simulink model "Kinematic_Model_Simulink"  (R2022a)
settings: Solver=ode14x  StartTime=0.0  StopTime=0.7  FixedStep=0.0005  RelTol=1e-3
values from neighbouring files (symbols this model uses):
  a_joint = 160/180*pi    (= 2.79252680319)    [Kinematic_Model_Activation.m]    (also in Kinematic_Model_sweep_double.m; Kinematic_Model_sweep_single.m)
  C_damping = 10    [Kinematic_Model_Activation.m]    (also in Kinematic_Model_sweep_double.m; Kinematic_Model_sweep_single.m = 100)
  g = [0;0;-9.81]    [Kinematic_Model_Activation.m]    (also in Kinematic_Model_sweep_double.m; Kinematic_Model_sweep_single.m)
  k_cable = 1200    [Kinematic_Model_Activation.m]    (also in Kinematic_Model_sweep_single.m)
  k_joint = 35    [Kinematic_Model_Activation.m]    (also in Kinematic_Model_sweep_double.m; Kinematic_Model_sweep_single.m)
  l_cable = sqrt(6)/4*l_leg*sin(a_joint/2)*(1 - delta)    [Kinematic_Model_Activation.m]    (also in Kinematic_Model_sweep_double.m; Kinematic_Model_sweep_single.m)
  l_leg = 0.3    [Kinematic_Model_Activation.m]    (also in Kinematic_Model_sweep_double.m; Kinematic_Model_sweep_single.m)
  m_bar = m_leg/2    (= 0.331383847657)    [Kinematic_Model_Activation.m]    (also in Kinematic_Model_sweep_double.m; Kinematic_Model_sweep_single.m)
  mu_k = 0.35    [Kinematic_Model_Activation.m]    (also in Kinematic_Model_sweep_double.m; Kinematic_Model_sweep_single.m)
  mu_s = 0.45    [Kinematic_Model_Activation.m]    (also in Kinematic_Model_sweep_double.m; Kinematic_Model_sweep_single.m)
  nu_s = 0.2    [Kinematic_Model_Activation.m]    (also in Kinematic_Model_sweep_double.m; Kinematic_Model_sweep_single.m)
  T_damping = 1    [Kinematic_Model_Activation.m]    (also in Kinematic_Model_sweep_double.m; Kinematic_Model_sweep_single.m)
(part 1 of 2)
settings Model: Creator=LZY-ALIENWARE15  LastModifiedBy=S2974177
settings SolverCC: ExtrapolationOrder=3  AlgebraicLoopSolver=TrustRegion
settings DebuggingCC: UnconnectedInputMsg=warning  UnconnectedOutputMsg=warning  UnconnectedLineMsg=warning  SFMachineParentedDataDiag=warning  UnderSpecifiedDimensionMsg=warning
settings RTWCC: DLArmComputeVersion=19.05

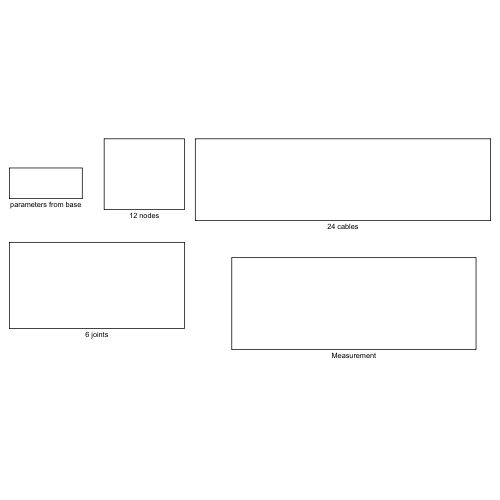
[thumbnail: Simulink's stored preview of the top-level diagram]
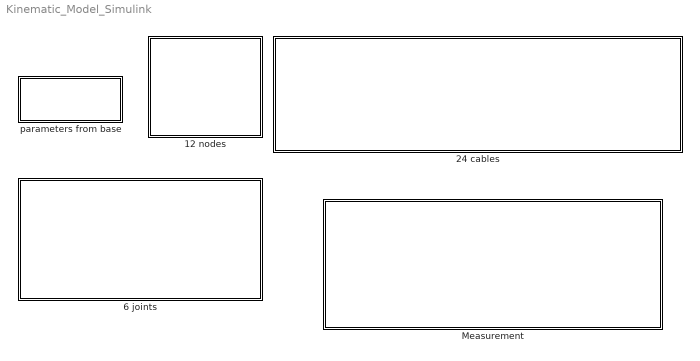
== system Kinematic_Model_Simulink ==
  "12 nodes " : Subsystem
  24 cables : Subsystem
  6 joints : Subsystem
  Measurement : Subsystem
  parameters from base : Subsystem

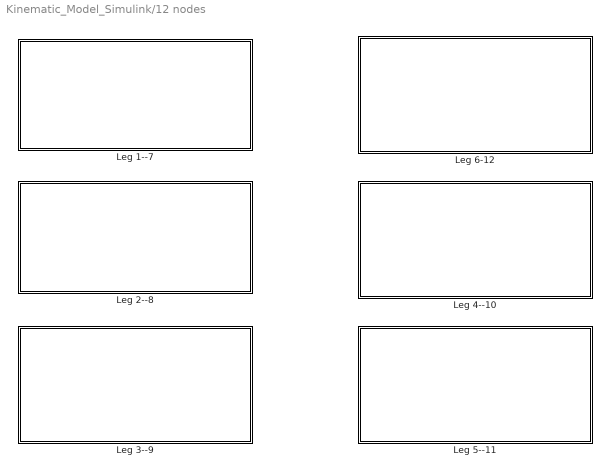
== system Kinematic_Model_Simulink/12 nodes  ==
  Leg 1--7 : Subsystem
  Leg 2--8 : Subsystem
  Leg 3--9 : Subsystem
  Leg 4--10 : Subsystem
  Leg 5--11 : Subsystem
  Leg 6-12 : Subsystem

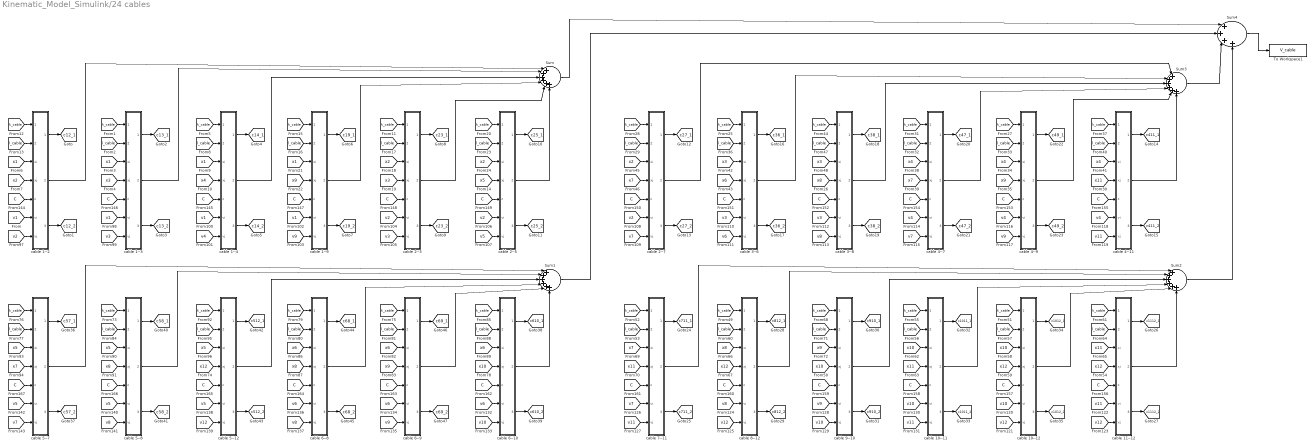
== system Kinematic_Model_Simulink/24 cables ==
  Sum{,1..3} (4 alike) : Sum  Inputs=|++++++
  Sum4 : Sum  Inputs=|++++
  To Workspace1 : ToWorkspace  VariableName=V_cable  SaveFormat=Timeseries  SampleTime=-1
  cable 1--2 : MATLAB Function  TreatAsAtomicUnit=on
  cable 1--3 : MATLAB Function  TreatAsAtomicUnit=on
  cable 1--4 : MATLAB Function  TreatAsAtomicUnit=on
  cable 1--9 : MATLAB Function  TreatAsAtomicUnit=on
  cable 10--11 : MATLAB Function  TreatAsAtomicUnit=on
  cable 10--12 : MATLAB Function  TreatAsAtomicUnit=on
  cable 11--12 : MATLAB Function  TreatAsAtomicUnit=on
  cable 2--3 : MATLAB Function  TreatAsAtomicUnit=on
  cable 2--5 : MATLAB Function  TreatAsAtomicUnit=on
  cable 2--7 : MATLAB Function  TreatAsAtomicUnit=on
  cable 3--6 : MATLAB Function  TreatAsAtomicUnit=on
  cable 3--8 : MATLAB Function  TreatAsAtomicUnit=on
  cable 4--11 : MATLAB Function  TreatAsAtomicUnit=on
  cable 4--7 : MATLAB Function  TreatAsAtomicUnit=on
  cable 4--9 : MATLAB Function  TreatAsAtomicUnit=on
  cable 5--12 : MATLAB Function  TreatAsAtomicUnit=on
  cable 5--7 : MATLAB Function  TreatAsAtomicUnit=on
  cable 5--8 : MATLAB Function  TreatAsAtomicUnit=on
  cable 6--10 : MATLAB Function  TreatAsAtomicUnit=on
  cable 6--8 : MATLAB Function  TreatAsAtomicUnit=on
  cable 6--9 : MATLAB Function  TreatAsAtomicUnit=on
  cable 7--11 : MATLAB Function  TreatAsAtomicUnit=on
  cable 8--12 : MATLAB Function  TreatAsAtomicUnit=on
  cable 9--10 : MATLAB Function  TreatAsAtomicUnit=on
  tag scope: c1011_1=global, c1011_2=global, c1012_1=global, c1012_2=global, c1112_1=global, c1112_2=global, c12_1=global, c12_2=global, c13_1=global, c13_2=global, c14_1=global, c14_2=global, c19_1=global, c19_2=global, c23_1=global, c23_2=global, c25_1=global, c25_2=global, c27_1=global, c27_2=global, c36_1=global, c36_2=global, c38_1=global, c38_2=global, c411_1=global, c411_2=global, c47_1=global, c47_2=global, c49_1=global, c49_2=global, c512_1=global, c512_2=global, c57_1=global, c57_2=global, c58_1=global, c58_2=global, c610_1=global, c610_2=global, c68_1=global, c68_2=global, c69_1=global, c69_2=global, c711_1=global, c711_2=global, c812_1=global, c812_2=global, c910_1=global, c910_2=global
  wires:
  [k_cable] -> cable 1--2/1(k_cable)
  [x1] -> cable 1--2/3(xi)
  [x2] -> cable 1--2/4(xj)
  cable 1--2/1(out_i) -> [c12_1]
  cable 1--2/3(out_j) -> [c12_2]
  [l_cable] -> cable 1--2/2(l_cable)
  [l_cable] -> cable 1--3/2(l_cable)
  [x1] -> cable 1--3/3(xi)
  [x3] -> cable 1--3/4(xj)
  cable 1--3/3(out_j) -> [c13_2]
  [k_cable] -> cable 1--3/1(k_cable)
  cable 1--3/1(out_i) -> [c13_1]
  [l_cable] -> cable 1--4/2(l_cable)
  [x1] -> cable 1--4/3(xi)
  [x4] -> cable 1--4/4(xj)
  cable 1--4/3(out_j) -> [c14_2]
  [k_cable] -> cable 1--4/1(k_cable)
  cable 1--4/1(out_i) -> [c14_1]
  [l_cable] -> cable 2--3/2(l_cable)
  [k_cable] -> cable 2--5/1(k_cable)
  cable 2--5/1(out_i) -> [c25_1]
  [x2] -> cable 2--5/3(xi)
  cable 2--5/3(out_j) -> [c25_2]
  cable 2--3/1(out_i) -> [c23_1]
  cable 2--3/3(out_j) -> [c23_2]
  [x3] -> cable 2--3/4(xj)
  [x1] -> cable 1--9/3(xi)
  [l_cable] -> cable 1--9/2(l_cable)
  [l_cable] -> cable 2--5/2(l_cable)
  [x9] -> cable 1--9/4(xj)
  [k_cable] -> cable 1--9/1(k_cable)
  [x2] -> cable 2--3/3(xi)
  cable 1--9/3(out_j) -> [c19_2]
  [k_cable] -> cable 2--3/1(k_cable)
  cable 1--9/1(out_i) -> [c19_1]
  [x5] -> cable 2--5/4(xj)
  [l_cable] -> cable 3--6/2(l_cable)
  [k_cable] -> cable 3--8/1(k_cable)
  cable 3--8/1(out_i) -> [c38_1]
  cable 3--8/3(out_j) -> [c38_2]
  cable 3--6/1(out_i) -> [c36_1]
  cable 3--6/3(out_j) -> [c36_2]
  [x6] -> cable 3--6/4(xj)
  [x7] -> cable 4--7/4(xj)
  [l_cable] -> cable 4--7/2(l_cable)
  [x4] -> cable 4--7/3(xi)
  [x9] -> cable 4--9/4(xj)
  cable 4--9/3(out_j) -> [c49_2]
  cable 4--11/3(out_j) -> [c411_2]
  [x4] -> cable 4--11/3(xi)
  [x11] -> cable 4--11/4(xj)
  cable 4--9/1(out_i) -> [c49_1]
  cable 4--7/1(out_i) -> [c47_1]
  [k_cable] -> cable 4--9/1(k_cable)
  cable 4--7/3(out_j) -> [c47_2]
  [k_cable] -> cable 4--7/1(k_cable)
  [x4] -> cable 4--9/3(xi)
  [x7] -> cable 2--7/4(xj)
  cable 2--7/3(out_j) -> [c27_2]
  [x3] -> cable 3--6/3(xi)
  [k_cable] -> cable 2--7/1(k_cable)
  [l_cable] -> cable 4--11/2(l_cable)
  cable 4--11/1(out_i) -> [c411_1]
  [x3] -> cable 3--8/3(xi)
  cable 2--7/1(out_i) -> [c27_1]
  [k_cable] -> cable 3--6/1(k_cable)
  [x8] -> cable 3--8/4(xj)
  [k_cable] -> cable 4--11/1(k_cable)
  [x2] -> cable 2--7/3(xi)
  [l_cable] -> cable 2--7/2(l_cable)
  [l_cable] -> cable 3--8/2(l_cable)
  [l_cable] -> cable 4--9/2(l_cable)
  [l_cable] -> cable 8--12/2(l_cable)
  [k_cable] -> cable 9--10/1(k_cable)
  cable 9--10/1(out_i) -> [c910_1]
  cable 9--10/3(out_j) -> [c910_2]
  cable 8--12/1(out_i) -> [c812_1]
  cable 8--12/3(out_j) -> [c812_2]
  [x12] -> cable 8--12/4(xj)
  [x11] -> cable 10--11/4(xj)
  [l_cable] -> cable 10--11/2(l_cable)
  [x10] -> cable 10--11/3(xi)
  [x12] -> cable 10--12/4(xj)
  cable 10--12/3(out_j) -> [c1012_2]
  cable 11--12/3(out_j) -> [c1112_2]
  [x11] -> cable 11--12/3(xi)
  [x12] -> cable 11--12/4(xj)
  cable 10--12/1(out_i) -> [c1012_1]
  cable 10--11/1(out_i) -> [c1011_1]
  [k_cable] -> cable 10--12/1(k_cable)
  cable 10--11/3(out_j) -> [c1011_2]
  [k_cable] -> cable 10--11/1(k_cable)
  [x10] -> cable 10--12/3(xi)
  [x11] -> cable 7--11/4(xj)
  cable 7--11/3(out_j) -> [c711_2]
  [x8] -> cable 8--12/3(xi)
  [k_cable] -> cable 7--11/1(k_cable)
  [l_cable] -> cable 11--12/2(l_cable)
  cable 11--12/1(out_i) -> [c1112_1]
  [x9] -> cable 9--10/3(xi)
  cable 7--11/1(out_i) -> [c711_1]
  [k_cable] -> cable 8--12/1(k_cable)
  [x10] -> cable 9--10/4(xj)
  [k_cable] -> cable 11--12/1(k_cable)
  [x7] -> cable 7--11/3(xi)
  [l_cable] -> cable 7--11/2(l_cable)
  [l_cable] -> cable 9--10/2(l_cable)
  [l_cable] -> cable 10--12/2(l_cable)
  [l_cable] -> cable 5--8/2(l_cable)
  [k_cable] -> cable 5--12/1(k_cable)
  cable 5--12/1(out_i) -> [c512_1]
  cable 5--12/3(out_j) -> [c512_2]
  cable 5--8/1(out_i) -> [c58_1]
  cable 5--8/3(out_j) -> [c58_2]
  [x8] -> cable 5--8/4(xj)
  [x8] -> cable 6--8/4(xj)
  [l_cable] -> cable 6--8/2(l_cable)
  [x6] -> cable 6--8/3(xi)
  [x9] -> cable 6--9/4(xj)
  cable 6--9/3(out_j) -> [c69_2]
  cable 6--10/3(out_j) -> [c610_2]
  [x6] -> cable 6--10/3(xi)
  [x10] -> cable 6--10/4(xj)
  cable 6--9/1(out_i) -> [c69_1]
  cable 6--8/1(out_i) -> [c68_1]
  [k_cable] -> cable 6--9/1(k_cable)
  cable 6--8/3(out_j) -> [c68_2]
  [k_cable] -> cable 6--8/1(k_cable)
  [x6] -> cable 6--9/3(xi)
  [x7] -> cable 5--7/4(xj)
  cable 5--7/3(out_j) -> [c57_2]
  [x5] -> cable 5--8/3(xi)
  [k_cable] -> cable 5--7/1(k_cable)
  [l_cable] -> cable 6--10/2(l_cable)
  cable 6--10/1(out_i) -> [c610_1]
  [x5] -> cable 5--12/3(xi)
  cable 5--7/1(out_i) -> [c57_1]
  [k_cable] -> cable 5--8/1(k_cable)
  [x12] -> cable 5--12/4(xj)
  [k_cable] -> cable 6--10/1(k_cable)
  [x5] -> cable 5--7/3(xi)
  [l_cable] -> cable 5--7/2(l_cable)
  [l_cable] -> cable 5--12/2(l_cable)
  [l_cable] -> cable 6--9/2(l_cable)
  cable 1--2/2(E_cable) -> Sum/1
  cable 10--11/2(E_cable) -> Sum2/4
  cable 9--10/2(E_cable) -> Sum2/3
  cable 10--12/2(E_cable) -> Sum2/5
  cable 11--12/2(E_cable) -> Sum2/6
  cable 8--12/2(E_cable) -> Sum2/2
  cable 7--11/2(E_cable) -> Sum2/1
  cable 6--10/2(E_cable) -> Sum1/6
  cable 6--9/2(E_cable) -> Sum1/5
  cable 6--8/2(E_cable) -> Sum1/4
  cable 5--12/2(E_cable) -> Sum1/3
  cable 5--8/2(E_cable) -> Sum1/2
  cable 5--7/2(E_cable) -> Sum1/1
  cable 1--3/2(E_cable) -> Sum/2
  cable 1--4/2(E_cable) -> Sum/3
  cable 1--9/2(E_cable) -> Sum/4
  cable 2--3/2(E_cable) -> Sum/5
  cable 2--5/2(E_cable) -> Sum/6
  cable 2--7/2(E_cable) -> Sum3/1
  cable 3--6/2(E_cable) -> Sum3/2
  cable 3--8/2(E_cable) -> Sum3/3
  cable 4--7/2(E_cable) -> Sum3/4
  cable 4--9/2(E_cable) -> Sum3/5
  cable 4--11/2(E_cable) -> Sum3/6
  Sum3/1 -> Sum4/3
  Sum2/1 -> Sum4/4
  Sum1/1 -> Sum4/2
  Sum/1 -> Sum4/1
  Sum4/1 -> To Workspace1/1
  [v1] -> cable 1--2/6(vi)
  [v2] -> cable 1--2/7(vj)
  [v4] -> cable 1--4/7(vj)
  [v1] -> cable 1--4/6(vi)
  [v1] -> cable 1--9/6(vi)
  [v9] -> cable 1--9/7(vj)
  [v1] -> cable 1--3/6(vi)
  [v3] -> cable 1--3/7(vj)
  [v2] -> cable 2--3/6(vi)
  [v3] -> cable 2--3/7(vj)
  [v2] -> cable 2--5/6(vi)
  [v5] -> cable 2--5/7(vj)
  [v2] -> cable 2--7/6(vi)
  [v7] -> cable 2--7/7(vj)
  [v3] -> cable 3--6/6(vi)
  [v6] -> cable 3--6/7(vj)
  [v3] -> cable 3--8/6(vi)
  [v8] -> cable 3--8/7(vj)
  [v4] -> cable 4--7/6(vi)
  [v7] -> cable 4--7/7(vj)
  [v4] -> cable 4--9/6(vi)
  [v9] -> cable 4--9/7(vj)
  [v4] -> cable 4--11/6(vi)
  [v11] -> cable 4--11/7(vj)
  [v10] -> cable 10--12/6(vi)
  [v12] -> cable 10--12/7(vj)
  [v11] -> cable 11--12/6(vi)
  [v12] -> cable 11--12/7(vj)
  [v8] -> cable 8--12/6(vi)
  [v12] -> cable 8--12/7(vj)
  [v7] -> cable 7--11/6(vi)
  [v11] -> cable 7--11/7(vj)
  [v9] -> cable 9--10/6(vi)
  [v10] -> cable 9--10/7(vj)
  [v10] -> cable 10--11/6(vi)
  [v11] -> cable 10--11/7(vj)
  [v6] -> cable 6--10/6(vi)
  [v10] -> cable 6--10/7(vj)
  [v6] -> cable 6--9/6(vi)
  [v9] -> cable 6--9/7(vj)
  [v6] -> cable 6--8/6(vi)
  [v8] -> cable 6--8/7(vj)
  [v5] -> cable 5--12/6(vi)
  [v12] -> cable 5--12/7(vj)
  [v5] -> cable 5--8/6(vi)
  [v8] -> cable 5--8/7(vj)
  [v5] -> cable 5--7/6(vi)
  [v7] -> cable 5--7/7(vj)
  [C] -> cable 1--2/5(c)
  [C] -> cable 1--4/5(c)
  [C] -> cable 1--3/5(c)
  [C] -> cable 1--9/5(c)
  [C] -> cable 2--3/5(c)
  [C] -> cable 2--5/5(c)
  [C] -> cable 2--7/5(c)
  [C] -> cable 3--6/5(c)
  [C] -> cable 3--8/5(c)
  [C] -> cable 4--9/5(c)
  [C] -> cable 4--7/5(c)
  [C] -> cable 4--11/5(c)
  [C] -> cable 11--12/5(c)
  [C] -> cable 10--12/5(c)
  [C] -> cable 10--11/5(c)
  [C] -> cable 9--10/5(c)
  [C] -> cable 8--12/5(c)
  [C] -> cable 7--11/5(c)
  [C] -> cable 6--10/5(c)
  [C] -> cable 6--9/5(c)
  [C] -> cable 6--8/5(c)
  [C] -> cable 5--12/5(c)
  [C] -> cable 5--8/5(c)
  [C] -> cable 5--7/5(c)

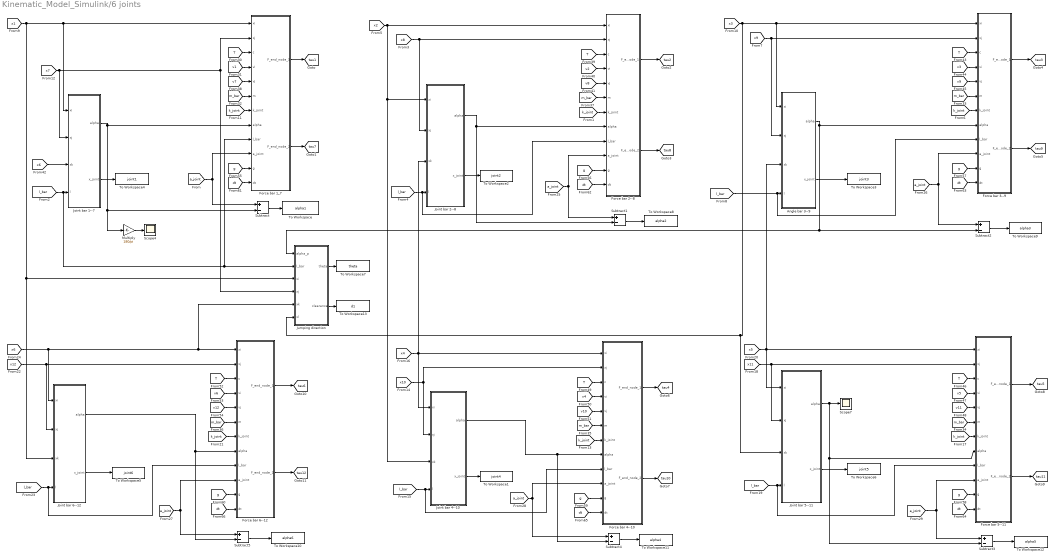
== system Kinematic_Model_Simulink/6 joints ==
  Angle bar 3--9 : MATLAB Function  TreatAsAtomicUnit=on
  Force bar 1_7 : MATLAB Function  TreatAsAtomicUnit=on
  Force bar 2--8 : MATLAB Function  TreatAsAtomicUnit=on
  Force bar 3--9 : MATLAB Function  TreatAsAtomicUnit=on
  Force bar 4--10 : MATLAB Function  TreatAsAtomicUnit=on
  Force bar 5--11 : MATLAB Function  TreatAsAtomicUnit=on
  Force bar 6--12 : MATLAB Function  TreatAsAtomicUnit=on
  Joint bar 1--7 : MATLAB Function  TreatAsAtomicUnit=on
  Joint bar 2--8 : MATLAB Function  TreatAsAtomicUnit=on
  Joint bar 4--10 : MATLAB Function  TreatAsAtomicUnit=on
  Joint bar 5--11 : MATLAB Function  TreatAsAtomicUnit=on
  Joint bar 6--12 : MATLAB Function  TreatAsAtomicUnit=on
  Jumping direction : MATLAB Function  TreatAsAtomicUnit=on
  Multiply : Gain  Gain=180/pi
  Scope4 : Scope
  Scope7 : Scope
  Subtract{,1..5} (6 alike) : Sum  Inputs=+-
  To Workspace : ToWorkspace  VariableName=alpha1  SaveFormat=Timeseries  SampleTime=-1
  To Workspace1 : ToWorkspace  VariableName=joint4  SaveFormat=Timeseries  SampleTime=-1
  To Workspace10 : ToWorkspace  VariableName=alpha6  SaveFormat=Timeseries  SampleTime=-1
  To Workspace11 : ToWorkspace  VariableName=alpha4  SaveFormat=Timeseries  SampleTime=-1
  To Workspace12 : ToWorkspace  VariableName=alpha5  SaveFormat=Timeseries  SampleTime=-1
  To Workspace13 : ToWorkspace  VariableName=d1  SaveFormat=Timeseries  SampleTime=-1
  To Workspace2 : ToWorkspace  VariableName=joint2  SaveFormat=Timeseries  SampleTime=-1
  To Workspace3 : ToWorkspace  VariableName=joint3  SaveFormat=Timeseries  SampleTime=-1
  To Workspace4 : ToWorkspace  VariableName=joint1  SaveFormat=Timeseries  SampleTime=-1
  To Workspace5 : ToWorkspace  VariableName=joint6  SaveFormat=Timeseries  SampleTime=-1
  To Workspace6 : ToWorkspace  VariableName=joint5  SaveFormat=Timeseries  SampleTime=-1
  To Workspace7 : ToWorkspace  VariableName=theta  SaveFormat=Timeseries  SampleTime=-1
  To Workspace8 : ToWorkspace  VariableName=alpha2  SaveFormat=Timeseries  SampleTime=-1
  To Workspace9 : ToWorkspace  VariableName=alpha3  SaveFormat=Timeseries  SampleTime=-1
  tag scope: tau10=global, tau11=global, tau12=global, tau1=global, tau2=global, tau3=global, tau4=global, tau5=global, tau6=global, tau7=global, tau8=global, tau9=global
  wires:
  [x1] -> Jumping direction/3(xi), Joint bar 6--12/3(xk), Joint bar 1--7/1(xi), Force bar 1_7/1(xi)
  [x7] -> Joint bar 1--7/2(xj), Jumping direction/4(xj), Force bar 1_7/2(xj)
  Joint bar 1--7/1(alpha) -> Subtract/2, Multiply/1, Force bar 1_7/8(alpha)
  Force bar 1_7/1(F_end_node_1) -> [tau1]
  [k_joint] -> Force bar 1_7/7(k_joint)
  [l_bar] -> Force bar 1_7/9(l_bar), Jumping direction/2(l_bar), Joint bar 1--7/4(l)
  Force bar 2--8/2(F_end_node_2) -> [tau8]
  [x2] -> Joint bar 2--8/1(xi), Joint bar 4--10/3(xk), Force bar 2--8/1(xi)
  [k_joint] -> Force bar 2--8/7(k_joint)
  [l_bar] -> Force bar 2--8/9(l_bar), Joint bar 2--8/4(l)
  Force bar 2--8/1(F_end_node_1) -> [tau2]
  [x8] -> Joint bar 2--8/2(xj), Force bar 2--8/2(xj)
  [l_bar] -> Force bar 3--9/9(l_bar), Angle bar 3--9/4(l)
  Force bar 3--9/2(F_end_node_2) -> [tau9]
  Force bar 3--9/1(F_end_node_1) -> [tau3]
  [x3] -> Jumping direction/6(xl), Joint bar 5--11/3(xk), Angle bar 3--9/1(xi), Force bar 3--9/1(xi)
  [k_joint] -> Force bar 3--9/7(k_joint)
  [x9] -> Angle bar 3--9/2(xj), Force bar 3--9/2(xj)
  [x10] -> Joint bar 4--10/2(xj), Force bar 4--10/2(xj)
  Force bar 4--10/2(F_end_node_2) -> [tau10]
  [x4] -> Force bar 4--10/1(xi), Joint bar 4--10/1(xi), Joint bar 2--8/3(xk)
  [k_joint] -> Force bar 4--10/7(k_joint)
  [l_bar] -> Force bar 4--10/9(l_bar), Joint bar 4--10/4(l)
  Force bar 4--10/1(F_end_node_1) -> [tau4]
  [l_bar] -> Force bar 5--11/9(l_bar), Joint bar 5--11/4(l)
  [k_joint] -> Force bar 5--11/7(k_joint)
  Force bar 5--11/1(F_end_node_1) -> [tau5]
  [x5] -> Force bar 5--11/1(xi), Joint bar 5--11/1(xi), Angle bar 3--9/3(xk)
  Force bar 5--11/2(F_end_node_2) -> [tau11]
  [x12] -> Joint bar 6--12/2(xj), Force bar 6--12/2(xj)
  [k_joint] -> Force bar 6--12/7(k_joint)
  Force bar 6--12/1(F_end_node_1) -> [tau6]
  [x6] -> Joint bar 6--12/1(xi), Jumping direction/5(xk), Force bar 6--12/1(xi)
  Force bar 6--12/2(F_end_node_2) -> [tau12]
  [a_joint] -> Force bar 1_7/10(a_joint), Subtract/1
  [a_joint] -> Subtract5/1, Force bar 6--12/10(a_joint)
  [x11] -> Joint bar 5--11/2(xj), Force bar 5--11/2(xj)
  Jumping direction/1(theta) -> To Workspace7/1
  Jumping direction/2(clearance) -> To Workspace13/1
  [a_joint] -> Subtract1/1, Force bar 2--8/10(a_joint)
  Subtract1/1 -> To Workspace8/1
  [a_joint] -> Subtract2/1, Force bar 3--9/10(a_joint)
  Subtract2/1 -> To Workspace9/1
  [a_joint] -> Subtract3/1, Force bar 5--11/10(a_joint)
  Subtract3/1 -> To Workspace12/1
  [a_joint] -> Subtract4/1, Force bar 4--10/10(a_joint)
  Subtract4/1 -> To Workspace11/1
  Joint bar 6--12/1(alpha) -> Subtract5/2, Force bar 6--12/8(alpha)
  [l_bar] -> Force bar 6--12/9(l_bar), Joint bar 6--12/4(l)
  Subtract5/1 -> To Workspace10/1
  [m_bar] -> Force bar 1_7/6(m)
  Force bar 1_7/2(F_end_node_2) -> [tau7]
  [m_bar] -> Force bar 3--9/6(m)
  [m_bar] -> Force bar 5--11/6(m)
  [m_bar] -> Force bar 4--10/6(m)
  [m_bar] -> Force bar 6--12/6(m)
  [m_bar] -> Force bar 2--8/6(m)
  Subtract/1 -> To Workspace/1
  Joint bar 2--8/2(x_joint) -> To Workspace2/1
  Joint bar 5--11/2(x_joint) -> To Workspace6/1
  Joint bar 4--10/2(x_joint) -> To Workspace1/1
  Joint bar 6--12/2(x_joint) -> To Workspace5/1
  Angle bar 3--9/2(x_joint) -> To Workspace3/1
  Joint bar 1--7/2(x_joint) -> To Workspace4/1
  [x6] -> Joint bar 1--7/3(xk)
  [T] -> Force bar 1_7/3(c)
  [v1] -> Force bar 1_7/4(vi)
  [v7] -> Force bar 1_7/5(vj)
  [T] -> Force bar 2--8/3(c)
  [v2] -> Force bar 2--8/4(vi)
  [v8] -> Force bar 2--8/5(vj)
  [v3] -> Force bar 3--9/4(vi)
  [T] -> Force bar 3--9/3(c)
  [v9] -> Force bar 3--9/5(vj)
  [T] -> Force bar 5--11/3(c)
  [v5] -> Force bar 5--11/4(vi)
  [v11] -> Force bar 5--11/5(vj)
  [T] -> Force bar 4--10/3(c)
  [v4] -> Force bar 4--10/4(vi)
  [v10] -> Force bar 4--10/5(vj)
  [T] -> Force bar 6--12/3(c)
  [v12] -> Force bar 6--12/5(vj)
  [v6] -> Force bar 6--12/4(vi)
  [g] -> Force bar 1_7/11(g)
  [g] -> Force bar 2--8/11(g)
  [g] -> Force bar 3--9/11(g)
  [g] -> Force bar 5--11/11(g)
  [g] -> Force bar 4--10/11(g)
  [g] -> Force bar 6--12/11(g)
  Joint bar 2--8/1(alpha) -> Subtract1/2, Force bar 2--8/8(alpha)
  Angle bar 3--9/1(alpha) -> Jumping direction/1(alpha_p), Subtract2/2, Force bar 3--9/8(alpha)
  Joint bar 5--11/1(alpha) -> Subtract3/2, Force bar 5--11/8(alpha), Scope7/1
  Joint bar 4--10/1(alpha) -> Subtract4/2, Force bar 4--10/8(alpha)
  Multiply/1 -> Scope4/1
  [dt] -> Force bar 1_7/12(dt)
  [dt] -> Force bar 2--8/12(dt)
  [dt] -> Force bar 3--9/12(dt)
  [dt] -> Force bar 5--11/12(dt)
  [dt] -> Force bar 4--10/12(dt)
  [dt] -> Force bar 6--12/12(dt)

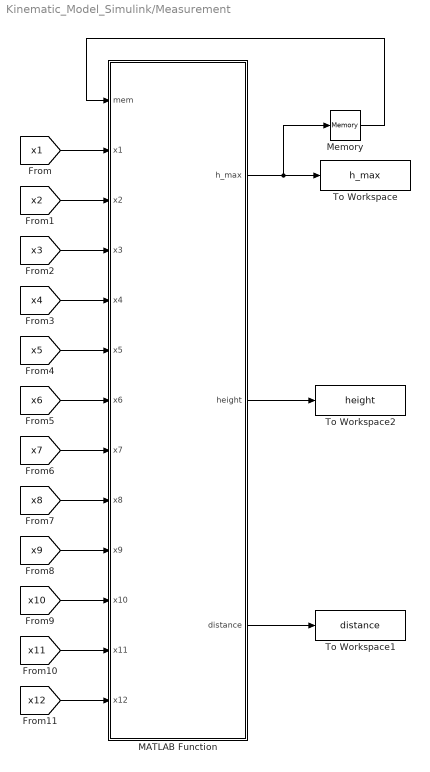
== system Kinematic_Model_Simulink/Measurement ==
  MATLAB Function : MATLAB Function  TreatAsAtomicUnit=on
  Memory : Memory
  To Workspace : ToWorkspace  VariableName=h_max  SaveFormat=Timeseries  SampleTime=-1
  To Workspace1 : ToWorkspace  VariableName=distance  SaveFormat=Timeseries  SampleTime=-1
  To Workspace2 : ToWorkspace  VariableName=height  SaveFormat=Timeseries  SampleTime=-1
  wires:
  [x1] -> MATLAB Function/2(x1)
  [x2] -> MATLAB Function/3(x2)
  [x3] -> MATLAB Function/4(x3)
  [x4] -> MATLAB Function/5(x4)
  [x5] -> MATLAB Function/6(x5)
  [x6] -> MATLAB Function/7(x6)
  [x8] -> MATLAB Function/9(x8)
  [x9] -> MATLAB Function/10(x9)
  [x10] -> MATLAB Function/11(x10)
  [x11] -> MATLAB Function/12(x11)
  [x12] -> MATLAB Function/13(x12)
  [x7] -> MATLAB Function/8(x7)
  MATLAB Function/3(distance) -> To Workspace1/1
  Memory/1 -> MATLAB Function/1(mem)
  MATLAB Function/1(h_max) -> Memory/1, To Workspace/1
  MATLAB Function/2(height) -> To Workspace2/1

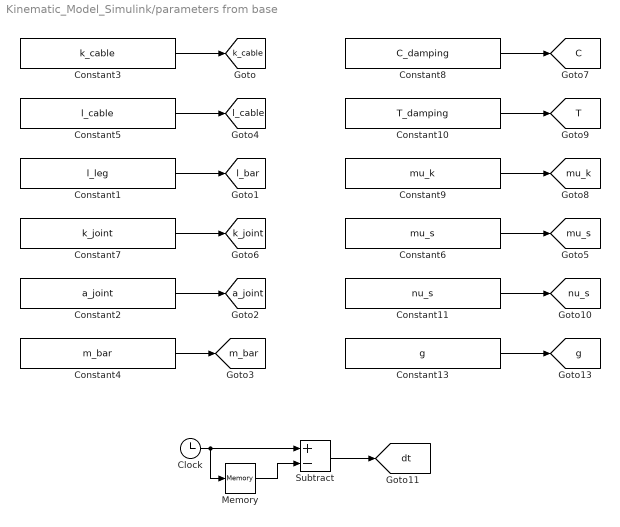
== system Kinematic_Model_Simulink/parameters from base ==
  Clock : Clock
  Constant1 : Constant  Value=l_leg
  Constant10 : Constant  Value=T_damping
  Constant11 : Constant  Value=nu_s
  Constant13 : Constant  Value=g
  Constant2 : Constant  Value=a_joint
  Constant3 : Constant  Value=k_cable
  Constant4 : Constant  Value=m_bar
  Constant5 : Constant  Value=l_cable
  Constant6 : Constant  Value=mu_s
  Constant7 : Constant  Value=k_joint
  Constant8 : Constant  Value=C_damping
  Constant9 : Constant  Value=mu_k
  Memory : Memory
  Subtract : Sum  Inputs=+-
  tag scope: C=global, T=global, a_joint=global, dt=global, g=global, k_cable=global, k_joint=global, l_bar=global, l_cable=global, m_bar=global, mu_k=global, mu_s=global, nu_s=global
  wires:
  Constant3/1 -> [k_cable]
  Constant1/1 -> [l_bar]
  Constant5/1 -> [l_cable]
  Constant7/1 -> [k_joint]
  Constant2/1 -> [a_joint]
  Constant4/1 -> [m_bar]
  Constant8/1 -> [C]
  Constant9/1 -> [mu_k]
  Constant10/1 -> [T]
  Constant6/1 -> [mu_s]
  Constant11/1 -> [nu_s]
  Subtract/1 -> [dt]
  Clock/1 -> Subtract/1, Memory/1
  Memory/1 -> Subtract/2
  Constant13/1 -> [g]

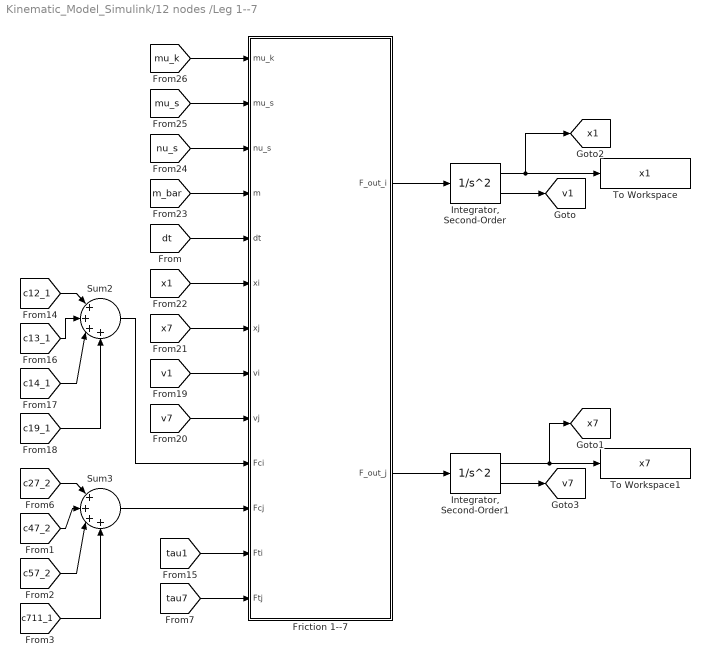
== system Kinematic_Model_Simulink/12 nodes /Leg 1--7 ==
  Friction 1--7 : MATLAB Function  TreatAsAtomicUnit=on
  "Integrator, Second-Order" : SecondOrderIntegrator  ICX=x1_ini  LimitX=on  LowerLimitX=[-inf;-inf;0]  ICDXDT=v1_ini
  "Integrator, Second-Order1" : SecondOrderIntegrator  ICX=x7_ini  LimitX=on  LowerLimitX=[-inf;-inf;0]  ICDXDT=[0;0;0]
  Sum2 : Sum  Inputs=|++++
  Sum3 : Sum  Inputs=|++++
  To Workspace : ToWorkspace  VariableName=x1  SaveFormat=Timeseries  SampleTime=-1
  To Workspace1 : ToWorkspace  VariableName=x7  SaveFormat=Timeseries  SampleTime=-1
  tag scope: v1=global, v7=global, x1=global, x7=global
  wires:
  "Integrator, Second-Order"/2 -> [v1]
  "Integrator, Second-Order1"/1 -> To Workspace1/1, [x7]
  "Integrator, Second-Order1"/2 -> [v7]
  [c14_1] -> Sum2/3
  [c19_1] -> Sum2/4
  [c13_1] -> Sum2/2
  [c12_1] -> Sum2/1
  [c57_2] -> Sum3/3
  [c47_2] -> Sum3/2
  [c711_1] -> Sum3/4
  [c27_2] -> Sum3/1
  Sum3/1 -> Friction 1--7/11(Fcj)
  Sum2/1 -> Friction 1--7/10(Fci)
  [v1] -> Friction 1--7/8(vi)
  [x7] -> Friction 1--7/7(xj)
  [x1] -> Friction 1--7/6(xi)
  [m_bar] -> Friction 1--7/4(m)
  [mu_k] -> Friction 1--7/1(mu_k)
  [mu_s] -> Friction 1--7/2(mu_s)
  [nu_s] -> Friction 1--7/3(nu_s)
  Friction 1--7/2(F_out_j) -> "Integrator, Second-Order1"/1
  [v7] -> Friction 1--7/9(vj)
  "Integrator, Second-Order"/1 -> [x1], To Workspace/1
  [dt] -> Friction 1--7/5(dt)
  Friction 1--7/1(F_out_i) -> "Integrator, Second-Order"/1
  [tau7] -> Friction 1--7/13(Ftj)
  [tau1] -> Friction 1--7/12(Fti)

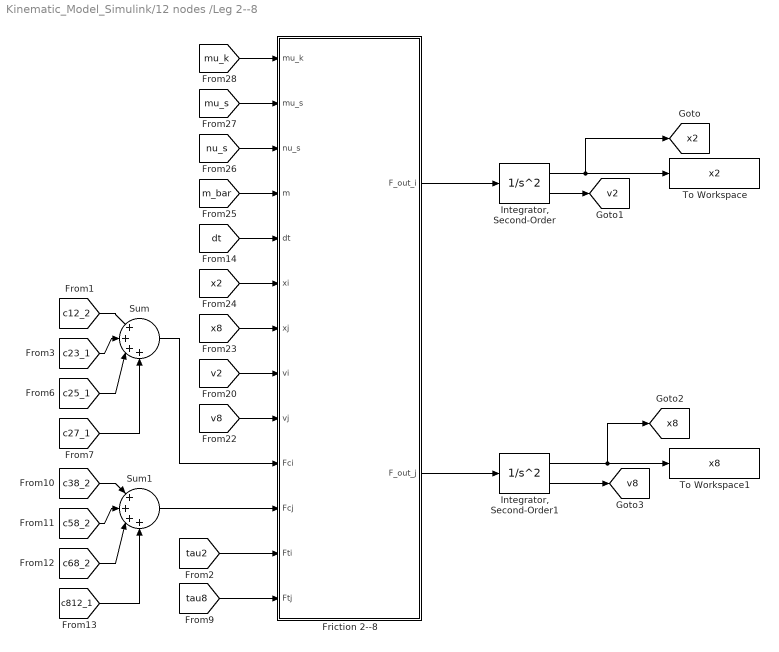
== system Kinematic_Model_Simulink/12 nodes /Leg 2--8 ==
  Friction 2--8 : MATLAB Function  TreatAsAtomicUnit=on
  "Integrator, Second-Order" : SecondOrderIntegrator  ICX=x2_ini  LimitX=on  LowerLimitX=[-inf;-inf;0]  ICDXDT=[0;0;0]
  "Integrator, Second-Order1" : SecondOrderIntegrator  ICX=x8_ini  LimitX=on  LowerLimitX=[-inf;-inf;0]  ICDXDT=[0;0;0]
  Sum : Sum  Inputs=|++++
  Sum1 : Sum  Inputs=|++++
  To Workspace : ToWorkspace  VariableName=x2  SaveFormat=Timeseries  SampleTime=-1
  To Workspace1 : ToWorkspace  VariableName=x8  SaveFormat=Timeseries  SampleTime=-1
  tag scope: v2=global, v8=global, x2=global, x8=global
  wires:
  "Integrator, Second-Order"/1 -> [x2], To Workspace/1
  "Integrator, Second-Order"/2 -> [v2]
  "Integrator, Second-Order1"/2 -> [v8]
  "Integrator, Second-Order1"/1 -> To Workspace1/1, [x8]
  [dt] -> Friction 2--8/5(dt)
  [v8] -> Friction 2--8/9(vj)
  [m_bar] -> Friction 2--8/4(m)
  [v2] -> Friction 2--8/8(vi)
  [mu_k] -> Friction 2--8/1(mu_k)
  [x8] -> Friction 2--8/7(xj)
  [x2] -> Friction 2--8/6(xi)
  [mu_s] -> Friction 2--8/2(mu_s)
  [nu_s] -> Friction 2--8/3(nu_s)
  [c23_1] -> Sum/2
  [c12_2] -> Sum/1
  [c25_1] -> Sum/3
  [c27_1] -> Sum/4
  Sum/1 -> Friction 2--8/10(Fci)
  [c812_1] -> Sum1/4
  [c68_2] -> Sum1/3
  [c58_2] -> Sum1/2
  [c38_2] -> Sum1/1
  Sum1/1 -> Friction 2--8/11(Fcj)
  Friction 2--8/2(F_out_j) -> "Integrator, Second-Order1"/1
  Friction 2--8/1(F_out_i) -> "Integrator, Second-Order"/1
  [tau8] -> Friction 2--8/13(Ftj)
  [tau2] -> Friction 2--8/12(Fti)

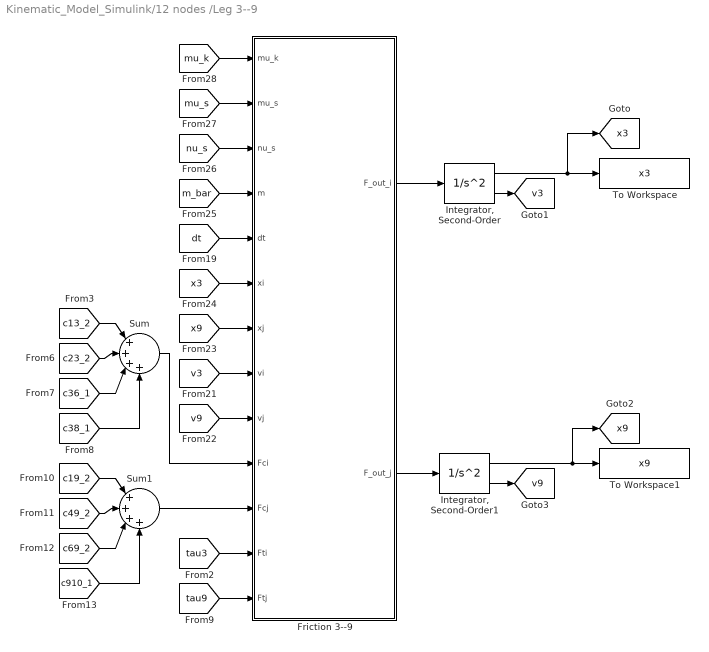
== system Kinematic_Model_Simulink/12 nodes /Leg 3--9 ==
  Friction 3--9 : MATLAB Function  TreatAsAtomicUnit=on
  "Integrator, Second-Order" : SecondOrderIntegrator  ICX=x3_ini  LimitX=on  LowerLimitX=[-inf;-inf;0]  ICDXDT=[0;0;0]
  "Integrator, Second-Order1" : SecondOrderIntegrator  ICX=x9_ini  LimitX=on  LowerLimitX=[-inf;-inf;0]  ICDXDT=[0;0;0]
  Sum : Sum  Inputs=|++++
  Sum1 : Sum  Inputs=|++++
  To Workspace : ToWorkspace  VariableName=x3  SaveFormat=Timeseries  SampleTime=-1
  To Workspace1 : ToWorkspace  VariableName=x9  SaveFormat=Timeseries  SampleTime=-1
  tag scope: v3=global, v9=global, x3=global, x9=global
  wires:
  "Integrator, Second-Order"/1 -> [x3], To Workspace/1
  "Integrator, Second-Order"/2 -> [v3]
  "Integrator, Second-Order1"/2 -> [v9]
  "Integrator, Second-Order1"/1 -> To Workspace1/1, [x9]
  [v3] -> Friction 3--9/8(vi)
  [nu_s] -> Friction 3--9/3(nu_s)
  [dt] -> Friction 3--9/5(dt)
  [v9] -> Friction 3--9/9(vj)
  [m_bar] -> Friction 3--9/4(m)
  [x3] -> Friction 3--9/6(xi)
  [mu_k] -> Friction 3--9/1(mu_k)
  [mu_s] -> Friction 3--9/2(mu_s)
  [x9] -> Friction 3--9/7(xj)
  [c38_1] -> Sum/4
  [c23_2] -> Sum/2
  [c13_2] -> Sum/1
  [c36_1] -> Sum/3
  Sum/1 -> Friction 3--9/10(Fci)
  [c49_2] -> Sum1/2
  [c69_2] -> Sum1/3
  [c19_2] -> Sum1/1
  [c910_1] -> Sum1/4
  Sum1/1 -> Friction 3--9/11(Fcj)
  Friction 3--9/2(F_out_j) -> "Integrator, Second-Order1"/1
  Friction 3--9/1(F_out_i) -> "Integrator, Second-Order"/1
  [tau3] -> Friction 3--9/12(Fti)
  [tau9] -> Friction 3--9/13(Ftj)

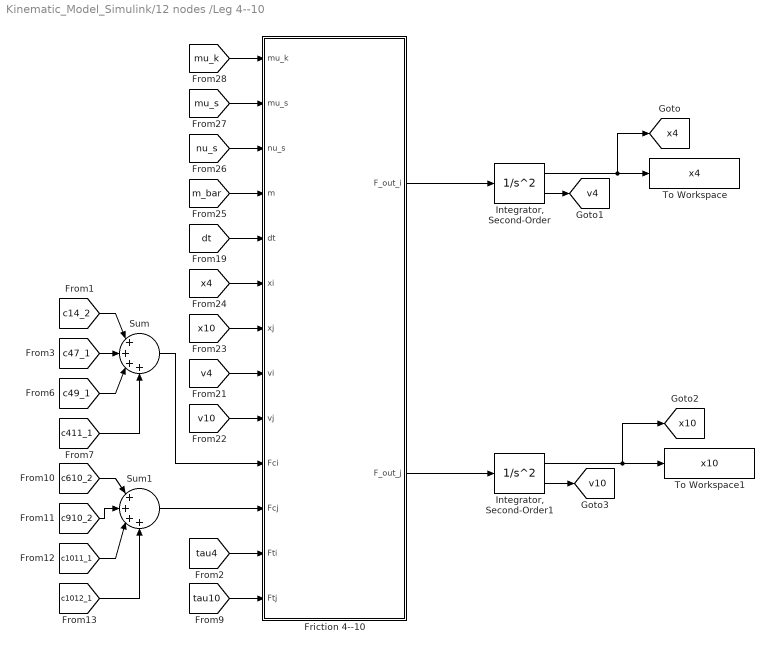
== system Kinematic_Model_Simulink/12 nodes /Leg 4--10 ==
  Friction 4--10 : MATLAB Function  TreatAsAtomicUnit=on
  "Integrator, Second-Order" : SecondOrderIntegrator  ICX=x4_ini  LimitX=on  LowerLimitX=[-inf;-inf;0]  ICDXDT=x4_ini
  "Integrator, Second-Order1" : SecondOrderIntegrator  ICX=x10_ini  LimitX=on  LowerLimitX=[-inf;-inf;0]  ICDXDT=[0;0;0]
  Sum : Sum  Inputs=|++++
  Sum1 : Sum  Inputs=|++++
  To Workspace : ToWorkspace  VariableName=x4  SaveFormat=Timeseries  SampleTime=-1
  To Workspace1 : ToWorkspace  VariableName=x10  SaveFormat=Timeseries  SampleTime=-1
  tag scope: v10=global, v4=global, x10=global, x4=global
  wires:
  "Integrator, Second-Order"/1 -> [x4], To Workspace/1
  "Integrator, Second-Order"/2 -> [v4]
  "Integrator, Second-Order1"/2 -> [v10]
  "Integrator, Second-Order1"/1 -> [x10], To Workspace1/1
  [nu_s] -> Friction 4--10/3(nu_s)
  [mu_s] -> Friction 4--10/2(mu_s)
  [x4] -> Friction 4--10/6(xi)
  [x10] -> Friction 4--10/7(xj)
  [mu_k] -> Friction 4--10/1(mu_k)
  [v4] -> Friction 4--10/8(vi)
  [m_bar] -> Friction 4--10/4(m)
  [dt] -> Friction 4--10/5(dt)
  [v10] -> Friction 4--10/9(vj)
  [c47_1] -> Sum/2
  [c411_1] -> Sum/4
  [c49_1] -> Sum/3
  [tau4] -> Friction 4--10/12(Fti)
  [c14_2] -> Sum/1
  Sum/1 -> Friction 4--10/10(Fci)
  [c910_2] -> Sum1/2
  [c1012_1] -> Sum1/4
  [c1011_1] -> Sum1/3
  [c610_2] -> Sum1/1
  [tau10] -> Friction 4--10/13(Ftj)
  Sum1/1 -> Friction 4--10/11(Fcj)
  Friction 4--10/2(F_out_j) -> "Integrator, Second-Order1"/1
  Friction 4--10/1(F_out_i) -> "Integrator, Second-Order"/1

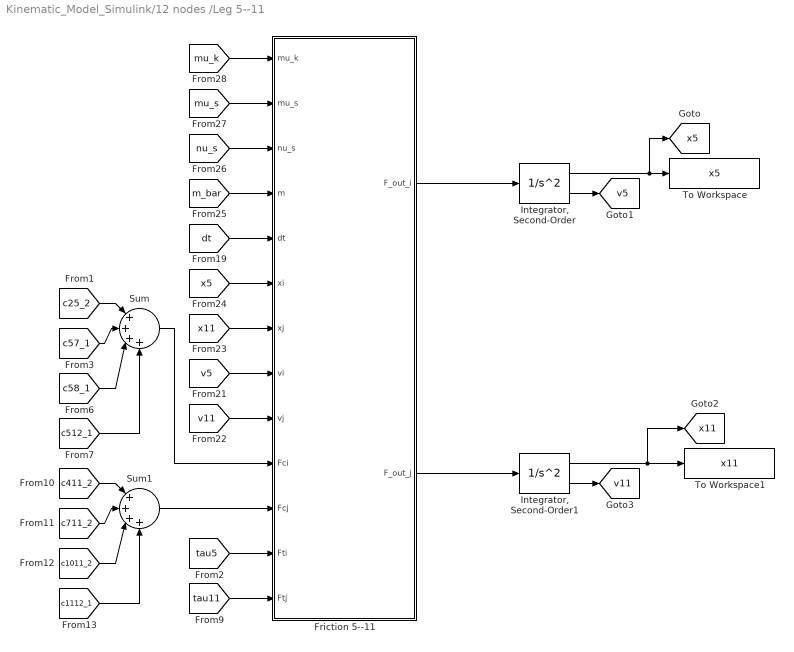
== system Kinematic_Model_Simulink/12 nodes /Leg 5--11 ==
  Friction 5--11 : MATLAB Function  TreatAsAtomicUnit=on
  "Integrator, Second-Order" : SecondOrderIntegrator  ICX=x5_ini  LimitX=on  LowerLimitX=[-inf;-inf;0]  ICDXDT=[0;0;0]
  "Integrator, Second-Order1" : SecondOrderIntegrator  ICX=x11_ini  LimitX=on  LowerLimitX=[-inf;-inf;0]  ICDXDT=[0;0;0]
  Sum : Sum  Inputs=|++++
  Sum1 : Sum  Inputs=|++++
  To Workspace : ToWorkspace  VariableName=x5  SaveFormat=Timeseries  SampleTime=-1
  To Workspace1 : ToWorkspace  VariableName=x11  SaveFormat=Timeseries  SampleTime=-1
  tag scope: v11=global, v5=global, x11=global, x5=global
  wires:
  "Integrator, Second-Order"/2 -> [v5]
  "Integrator, Second-Order"/1 -> [x5], To Workspace/1
  "Integrator, Second-Order1"/1 -> [x11], To Workspace1/1
  "Integrator, Second-Order1"/2 -> [v11]
  [x11] -> Friction 5--11/7(xj)
  [dt] -> Friction 5--11/5(dt)
  [m_bar] -> Friction 5--11/4(m)
  [mu_k] -> Friction 5--11/1(mu_k)
  [v5] -> Friction 5--11/8(vi)
  [nu_s] -> Friction 5--11/3(nu_s)
  [v11] -> Friction 5--11/9(vj)
  [x5] -> Friction 5--11/6(xi)
  [mu_s] -> Friction 5--11/2(mu_s)
  [c58_1] -> Sum/3
  [c57_1] -> Sum/2
  [c512_1] -> Sum/4
  [c25_2] -> Sum/1
  [c1011_2] -> Sum1/3
  [c1112_1] -> Sum1/4
  [c711_2] -> Sum1/2
  [c411_2] -> Sum1/1
  Sum/1 -> Friction 5--11/10(Fci)
  Sum1/1 -> Friction 5--11/11(Fcj)
  Friction 5--11/2(F_out_j) -> "Integrator, Second-Order1"/1
  Friction 5--11/1(F_out_i) -> "Integrator, Second-Order"/1
  [tau5] -> Friction 5--11/12(Fti)
  [tau11] -> Friction 5--11/13(Ftj)

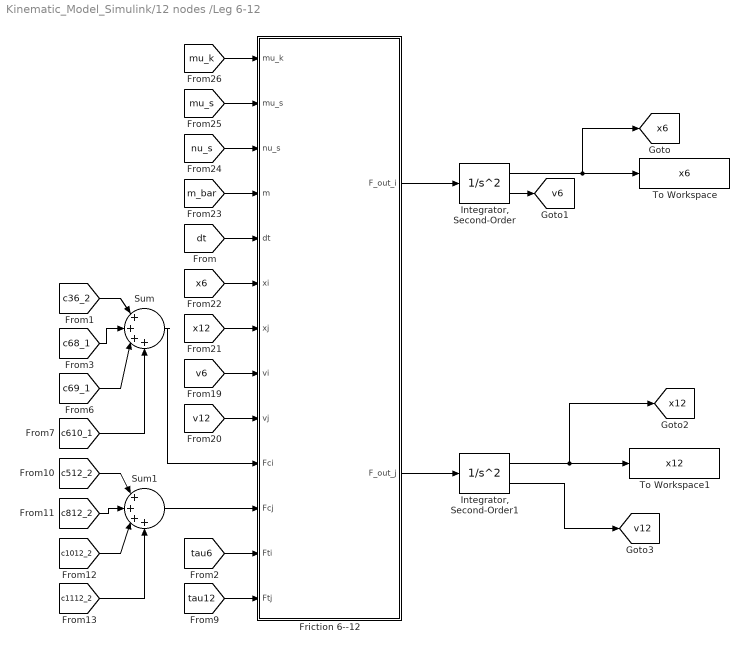
== system Kinematic_Model_Simulink/12 nodes /Leg 6-12 ==
  Friction 6--12 : MATLAB Function  TreatAsAtomicUnit=on
  "Integrator, Second-Order" : SecondOrderIntegrator  ICX=x6_ini  LimitX=on  LowerLimitX=[-inf;-inf;0]  ICDXDT=[0;0;0]
  "Integrator, Second-Order1" : SecondOrderIntegrator  ICX=x12_ini  LimitX=on  LowerLimitX=[-inf;-inf;0]  ICDXDT=[0;0;0]
  Sum : Sum  Inputs=|++++
  Sum1 : Sum  Inputs=|++++
  To Workspace : ToWorkspace  VariableName=x6  SaveFormat=Timeseries  SampleTime=-1
  To Workspace1 : ToWorkspace  VariableName=x12  SaveFormat=Timeseries  SampleTime=-1
  tag scope: v12=global, v6=global, x12=global, x6=global
  wires:
  "Integrator, Second-Order"/1 -> [x6], To Workspace/1
  "Integrator, Second-Order"/2 -> [v6]
  "Integrator, Second-Order1"/2 -> [v12]
  "Integrator, Second-Order1"/1 -> To Workspace1/1, [x12]
  [x6] -> Friction 6--12/6(xi)
  [x12] -> Friction 6--12/7(xj)
  [mu_k] -> Friction 6--12/1(mu_k)
  [m_bar] -> Friction 6--12/4(m)
  [v12] -> Friction 6--12/9(vj)
  [mu_s] -> Friction 6--12/2(mu_s)
  [v6] -> Friction 6--12/8(vi)
  [nu_s] -> Friction 6--12/3(nu_s)
  [c68_1] -> Sum/2
  [c69_1] -> Sum/3
  [c610_1] -> Sum/4
  [c36_2] -> Sum/1
  Sum/1 -> Friction 6--12/10(Fci)
  [c1112_2] -> Sum1/4
  [c1012_2] -> Sum1/3
  [c512_2] -> Sum1/1
  [c812_2] -> Sum1/2
  Sum1/1 -> Friction 6--12/11(Fcj)
  Friction 6--12/2(F_out_j) -> "Integrator, Second-Order1"/1
  Friction 6--12/1(F_out_i) -> "Integrator, Second-Order"/1
  [dt] -> Friction 6--12/5(dt)
  [tau12] -> Friction 6--12/13(Ftj)
  [tau6] -> Friction 6--12/12(Fti)

== matlab function Kinematic_Model_Simulink/12 nodes /Leg 2--8/Friction 2--8 ==
  data: mu_k input; F_out_i output; mu_s input; nu_s input; m input; dt input; xi input; xj input; vi input; vj input; Fci input; Fcj input; F_out_j output; Fti input; Ftj input
function [F_out_i, F_out_j] = ground_friction(mu_k, mu_s, nu_s, m, dt, xi, xj, vi, vj, Fci, Fcj, Fti, Ftj)
F_fi = [0;0;0];
F_fj = [0;0;0];

F_ni = [0;0;0];
F_nj = [0;0;0];
%% Friction modelling: Stribeck
% Fc: Coulomb Friction
% Fs: Static Friction
% 
% If node i touches the ground the following if-loop will commence
if  xi(3) <= 0 && dt~= 0
    F_ni = [0; 0; -Fti(3)-Fci(3)] - [0; 0; m*vi(3)/dt]; % Normal force with the ground
    if F_ni(3) > 0
        F_c = mu_k*norm(F_ni); % Coulomb term
        F_s = mu_s*norm(F_ni); % Static term
        F_fi = -(F_c + (F_s-F_c)*exp(-(norm(vi)/nu_s)^2))*signum(vi) + F_ni; % Sum of frictional and normal forces on node i
    end
end
% If node j touches the ground the following if-loop will commence
if xj(3) <= 0 && dt~= 0
    F_nj = [0; 0; -Ftj(3)-Fcj(3)] - [0; 0; m*vj(3)/dt]; % Normal force with the ground
    if F_nj(3) > 0
        F_c = mu_k*norm(F_nj); % Coulomb term
        F_s = mu_s*norm(F_nj); % Static term
        F_fj = -(F_c + (F_s-F_c)*exp(-(norm(vj)/nu_s)^2))*signum(vj) + F_nj; % Sum of frictional and normal forces on node j
    end
end


F_out_i = Fci + Fti + F_fi;
F_out_j = Fcj + Ftj + F_fj;



end

== matlab function Kinematic_Model_Simulink/Measurement/MATLAB Function ==
  data: h_max output; mem input; x1 input; height output; x2 input; x3 input; x4 input; x5 input; x6 input; x7 input; x8 input; x9 input; x10 input; x11 input; x12 input; distance output
function [h_max,height,distance] = measurement(mem,x1,x2,x3,x4,x5,x6,x7,x8,x9,x10,x11,x12)
xz = [x1(3) x2(3) x3(3) x4(3) x5(3) x6(3) x7(3) x8(3) x9(3) x10(3) x11(3) x12(3)];
height = min(xz);
if height > mem
    h_max = height;
else
    h_max = mem;
end

plane_pos = [x1(1:2) x2(1:2) x3(1:2) x4(1:2) x5(1:2) x6(1:2) x7(1:2) x8(1:2) x9(1:2) x10(1:2) x11(1:2) x12(1:2)];

distance = norm([sum(plane_pos(1,:))/12 ; sum(plane_pos(2,:))/12]);

end

== matlab function Kinematic_Model_Simulink/6 joints/Jumping direction ==
  data: alpha_p input; l_bar input; xi input; xj input; xk input; xl input; theta output; clearance output
function [theta, clearance] = Jump_Direction(alpha_p, l_bar, xi, xj, xk, xl)
% Transposes
nxi = transpose(xi);
nxj = transpose(xj);
nxk = transpose(xk);
nxl = transpose(xl);

% Normal vector
normal1 = cross(nxi-nxj, nxi-nxk);
normal2 = cross(nxi-nxl, nxi-nxk);

% Normalized
N1 = normal1/norm(normal1);
N2 = normal2/norm(normal2);

% Caclulation of jumping direction
CosTheta = max(min(dot(N2,N1)/(norm(N2)*norm(N1)),1),-1);
theta = real(acos(CosTheta));

% Calculation of lowest joint distance to ground (leg 3)
clearance = l_bar*sin(alpha_p/2 - theta);

end

== matlab function Kinematic_Model_Simulink/6 joints/Joint bar 1--7 ==
  data: xi input; alpha output; xj input; xk input; l input; x_joint output
function [alpha, x_joint]  = angle(xi, xj, xk, l)
%% Calculating the angle
d = norm(xi - xj); % Nodal distance
mag = (l^2-2*d^2)/l^2; % Term inside the inverse cosine to calculate the angle

if mag > -cos(160*pi/180)
    mag = -cos(160*pi/180);
    alpha = acos(mag);
else
    alpha = acos(mag);
end 
alpha*180/pi;
%% Plotting the Joint
% Distance from axis
d = l/2*cos(alpha/2);

% Vectors used for determination of the normal vector
nxi = transpose(xi);
nxj = transpose(xj);
nxk = transpose(xk);

% Normal vector of a plane created by a set of 2 parallel bars
normal = cross(nxi-nxj, nxi-nxk);
N = normal/norm(normal);

% Vector along the line between bar-connected nodes
x = nxj - nxi;
X = x/norm(x);

% Vector pointing outwards 
V = rotVec(X,N,-90);

% Position vector of the joint, to be used for plotting
x_joint = transpose(d*V + (nxj+nxi)/2);

end

== matlab function Kinematic_Model_Simulink/6 joints/Force bar 1_7 ==
  data: F_end_node_1 output; xi input; xj input; c input; vi input; vj input; m input; k_joint input; alpha input; l_bar input; a_joint input; F_end_node_2 output; g input; dt input
function [F_end_node_1, F_end_node_2]= Force(xi, xj, c, vi, vj, m, k_joint, alpha, l_bar, a_joint, g,dt)
% End node distance
x = xj - xi;
dist = norm(x);

% relative velocity of the two nodes w.r.t. each other
v = vj - vi;

% Torsion spring force and damping force
damp = -2*c*dot(x,v) / sqrt(dist^2*(l_bar^2 - dist^2)) * x/dist;
% Torsion spring force and damping force
if alpha < a_joint
    F_torsion = 1/2 * k_joint * (a_joint - alpha) / (cos(alpha/2)*l_bar/2);  
else
    F_torsion = - m/2*norm(v)/dt;
end

% Gravitational force
Fg_j = g/2;

% Calculation of the two parts of the torsion
F_end_node_1 = F_torsion *(-x)/dist - damp + Fg_j;
F_end_node_2 = F_torsion *x/dist + damp + Fg_j;

end

== matlab function Kinematic_Model_Simulink/12 nodes /Leg 4--10/Friction 4--10 ==
  data: mu_k input; F_out_i output; mu_s input; nu_s input; m input; dt input; xi input; xj input; vi input; vj input; Fci input; Fcj input; F_out_j output; Fti input; Ftj input
function [F_out_i, F_out_j] = ground_friction(mu_k, mu_s, nu_s, m, dt, xi, xj, vi, vj, Fci, Fcj, Fti, Ftj)
F_fi = [0;0;0];
F_fj = [0;0;0];

F_ni = [0;0;0];
F_nj = [0;0;0];
%% Friction modelling: Stribeck
% Fc: Coulomb Friction
% Fs: Static Friction
% 
% If node i touches the ground the following if-loop will commence
if  xi(3) <= 0 && dt~= 0
    F_ni = [0; 0; -Fti(3)-Fci(3)] - [0; 0; m*vi(3)/dt]; % Normal force with the ground
    if F_ni(3) > 0
        F_c = mu_k*norm(F_ni); % Coulomb term
        F_s = mu_s*norm(F_ni); % Static term
        F_fi = -(F_c + (F_s-F_c)*exp(-(norm(vi)/nu_s)^2))*signum(vi) + F_ni; % Sum of frictional and normal forces on node i
        
    end
end
% If node j touches the ground the following if-loop will commence
if xj(3) <= 0 && dt~= 0
    F_nj = [0; 0; -Ftj(3)-Fcj(3)] - [0; 0; m*vj(3)/dt]; % Normal force with the ground
    if F_nj(3) > 0
        F_c = mu_k*norm(F_nj); % Coulomb term
        F_s = mu_s*norm(F_nj); % Static term
        F_fj = -(F_c + (F_s-F_c)*exp(-(norm(vj)/nu_s)^2))*signum(vj) + F_nj; % Sum of frictional and normal forces on node j
    end
end


F_out_i = Fci + Fti + F_fi;
F_out_j = Fcj + Ftj + F_fj;



end

== matlab function Kinematic_Model_Simulink/24 cables/cable 1--9 ==
  data: out_i output; E_cable output; out_j output; k_cable input; l_cable input; xi input; xj input; c input; vi input; vj input
function [out_i, E_cable, out_j]= cable(k_cable,l_cable,xi,xj,c,vi,vj)
% damp and D are initialized as zero
damp = 0;
D = 0;

% Node distance
x = xj-xi;
dist = norm(x);

% Only when the cable is in tension there is non-zero force and damping
if  dist-l_cable > 0
    D = dist-l_cable;
    v = vj - vi;
    damp = -c*dot(v,x)/dist^2;
end

% Forces on the end nodes
out_i = k_cable*D*(x)/dist - damp*(x);
out_j = -k_cable*D*(x)/dist + damp*(x);

% Energy stored in the cable
E_cable = 0.5*k_cable*D^2;
end

== matlab function Kinematic_Model_Simulink/24 cables/cable 2--5 ==
  data: out_i output; E_cable output; out_j output; k_cable input; l_cable input; xi input; xj input; c input; vi input; vj input
function [out_i, E_cable, out_j]= cable(k_cable,l_cable,xi,xj,c,vi,vj)
% damp and D are initialized as zero
damp = 0;
D = 0;

% Node distance
x = xj-xi;
dist = norm(x);

% Only when the cable is in tension there is non-zero force and damping
if  dist-l_cable > 0
    D = dist-l_cable;
    v = vj - vi;
    damp = -c*dot(v,x)/dist^2;
end

% Forces on the end nodes
out_i = k_cable*D*(x)/dist - damp*(x);
out_j = -k_cable*D*(x)/dist + damp*(x);

% Energy stored in the cable
E_cable = 0.5*k_cable*D^2;
end

== matlab function Kinematic_Model_Simulink/24 cables/cable 4--9 ==
  data: out_i output; E_cable output; out_j output; k_cable input; l_cable input; xi input; xj input; c input; vi input; vj input
function [out_i, E_cable, out_j]= cable(k_cable,l_cable,xi,xj,c,vi,vj)
% damp and D are initialized as zero
damp = 0;
D = 0;

% Node distance
x = xj-xi;
dist = norm(x);

% Only when the cable is in tension there is non-zero force and damping
if  dist-l_cable > 0
    D = dist-l_cable;
    v = vj - vi;
    damp = -c*dot(v,x)/dist^2;
end

% Forces on the end nodes
out_i = k_cable*D*(x)/dist - damp*(x);
out_j = -k_cable*D*(x)/dist + damp*(x);

% Energy stored in the cable
E_cable = 0.5*k_cable*D^2;
end

== matlab function Kinematic_Model_Simulink/24 cables/cable 4--7 ==
  data: out_i output; E_cable output; out_j output; k_cable input; l_cable input; xi input; xj input; c input; vi input; vj input
function [out_i, E_cable, out_j]= cable(k_cable,l_cable,xi,xj,c,vi,vj)
% damp and D are initialized as zero
damp = 0;
D = 0;

% Node distance
x = xj-xi;
dist = norm(x);

% Only when the cable is in tension there is non-zero force and damping
if  dist-l_cable > 0
    D = dist-l_cable;
    v = vj - vi;
    damp = -c*dot(v,x)/dist^2;
end

% Forces on the end nodes
out_i = k_cable*D*(x)/dist - damp*(x);
out_j = -k_cable*D*(x)/dist + damp*(x);

% Energy stored in the cable
E_cable = 0.5*k_cable*D^2;
end

== matlab function Kinematic_Model_Simulink/24 cables/cable 4--11 ==
  data: out_i output; E_cable output; out_j output; k_cable input; l_cable input; xi input; xj input; c input; vi input; vj input
function [out_i, E_cable, out_j]= cable(k_cable,l_cable,xi,xj,c,vi,vj)
% damp and D are initialized as zero
damp = 0;
D = 0;

% Node distance
x = xj-xi;
dist = norm(x);

% Only when the cable is in tension there is non-zero force and damping
if  dist-l_cable > 0
    D = dist-l_cable;
    v = vj - vi;
    damp = -c*dot(v,x)/dist^2;
end

% Forces on the end nodes
out_i = k_cable*D*(x)/dist - damp*(x);
out_j = -k_cable*D*(x)/dist + damp*(x);

% Energy stored in the cable
E_cable = 0.5*k_cable*D^2;
end

== matlab function Kinematic_Model_Simulink/24 cables/cable 3--6 ==
  data: out_i output; E_cable output; out_j output; k_cable input; l_cable input; xi input; xj input; c input; vi input; vj input
function [out_i, E_cable, out_j]= cable(k_cable,l_cable,xi,xj,c,vi,vj)
% damp and D are initialized as zero
damp = 0;
D = 0;

% Node distance
x = xj-xi;
dist = norm(x);

% Only when the cable is in tension there is non-zero force and damping
if  dist-l_cable > 0
    D = dist-l_cable;
    v = vj - vi;
    damp = -c*dot(v,x)/dist^2;
end

% Forces on the end nodes
out_i = k_cable*D*(x)/dist - damp*(x);
out_j = -k_cable*D*(x)/dist + damp*(x);

% Energy stored in the cable
E_cable = 0.5*k_cable*D^2;
end

== matlab function Kinematic_Model_Simulink/24 cables/cable 2--7 ==
  data: out_i output; E_cable output; out_j output; k_cable input; l_cable input; xi input; xj input; c input; vi input; vj input
function [out_i, E_cable, out_j]= cable(k_cable,l_cable,xi,xj,c,vi,vj)
% damp and D are initialized as zero
damp = 0;
D = 0;

% Node distance
x = xj-xi;
dist = norm(x);

% Only when the cable is in tension there is non-zero force and damping
if  dist-l_cable > 0
    D = dist-l_cable;
    v = vj - vi;
    damp = -c*dot(v,x)/dist^2;
end

% Forces on the end nodes
out_i = k_cable*D*(x)/dist - damp*(x);
out_j = -k_cable*D*(x)/dist + damp*(x);

% Energy stored in the cable
E_cable = 0.5*k_cable*D^2;
end

== matlab function Kinematic_Model_Simulink/24 cables/cable 3--8 ==
  data: out_i output; E_cable output; out_j output; k_cable input; l_cable input; xi input; xj input; c input; vi input; vj input
function [out_i, E_cable, out_j]= cable(k_cable,l_cable,xi,xj,c,vi,vj)
% damp and D are initialized as zero
damp = 0;
D = 0;

% Node distance
x = xj-xi;
dist = norm(x);

% Only when the cable is in tension there is non-zero force and damping
if  dist-l_cable > 0
    D = dist-l_cable;
    v = vj - vi;
    damp = -c*dot(v,x)/dist^2;
end

% Forces on the end nodes
out_i = k_cable*D*(x)/dist - damp*(x);
out_j = -k_cable*D*(x)/dist + damp*(x);

% Energy stored in the cable
E_cable = 0.5*k_cable*D^2;
end

== matlab function Kinematic_Model_Simulink/24 cables/cable 1--3 ==
  data: out_i output; E_cable output; out_j output; k_cable input; l_cable input; xi input; xj input; c input; vi input; vj input
function [out_i, E_cable, out_j]= cable(k_cable,l_cable,xi,xj,c,vi,vj)
% damp and D are initialized as zero
damp = 0;
D = 0;

% Node distance
x = xj-xi;
dist = norm(x);

% Only when the cable is in tension there is non-zero force and damping
if  dist-l_cable > 0
    D = dist-l_cable;
    v = vj - vi;
    damp = -c*dot(v,x)/dist^2;
end

% Forces on the end nodes
out_i = k_cable*D*(x)/dist - damp*(x);
out_j = -k_cable*D*(x)/dist + damp*(x);

% Energy stored in the cable
E_cable = 0.5*k_cable*D^2;
end

== matlab function Kinematic_Model_Simulink/24 cables/cable 8--12 ==
  data: out_i output; E_cable output; out_j output; k_cable input; l_cable input; xi input; xj input; c input; vi input; vj input
function [out_i, E_cable, out_j]= cable(k_cable,l_cable,xi,xj,c,vi,vj)
% damp and D are initialized as zero
damp = 0;
D = 0;

% Node distance
x = xj-xi;
dist = norm(x);

% Only when the cable is in tension there is non-zero force and damping
if  dist-l_cable > 0
    D = dist-l_cable;
    v = vj - vi;
    damp = -c*dot(v,x)/dist^2;
end

% Forces on the end nodes
out_i = k_cable*D*(x)/dist - damp*(x);
out_j = -k_cable*D*(x)/dist + damp*(x);

% Energy stored in the cable
E_cable = 0.5*k_cable*D^2;
end

== matlab function Kinematic_Model_Simulink/24 cables/cable 7--11 ==
  data: out_i output; E_cable output; out_j output; k_cable input; l_cable input; xi input; xj input; c input; vi input; vj input
function [out_i, E_cable, out_j]= cable(k_cable,l_cable,xi,xj,c,vi,vj)
% damp and D are initialized as zero
damp = 0;
D = 0;

% Node distance
x = xj-xi;
dist = norm(x);

% Only when the cable is in tension there is non-zero force and damping
if  dist-l_cable > 0
    D = dist-l_cable;
    v = vj - vi;
    damp = -c*dot(v,x)/dist^2;
end

% Forces on the end nodes
out_i = k_cable*D*(x)/dist - damp*(x);
out_j = -k_cable*D*(x)/dist + damp*(x);

% Energy stored in the cable
E_cable = 0.5*k_cable*D^2;
end

== matlab function Kinematic_Model_Simulink/24 cables/cable 9--10 ==
  data: out_i output; E_cable output; out_j output; k_cable input; l_cable input; xi input; xj input; c input; vi input; vj input
function [out_i, E_cable, out_j]= cable(k_cable,l_cable,xi,xj,c,vi,vj)
% damp and D are initialized as zero
damp = 0;
D = 0;

% Node distance
x = xj-xi;
dist = norm(x);

% Only when the cable is in tension there is non-zero force and damping
if  dist-l_cable > 0
    D = dist-l_cable;
    v = vj - vi;
    damp = -c*dot(v,x)/dist^2;
end

% Forces on the end nodes
out_i = k_cable*D*(x)/dist - damp*(x);
out_j = -k_cable*D*(x)/dist + damp*(x);

% Energy stored in the cable
E_cable = 0.5*k_cable*D^2;
end

== matlab function Kinematic_Model_Simulink/24 cables/cable 10--12 ==
  data: out_i output; E_cable output; out_j output; k_cable input; l_cable input; xi input; xj input; c input; vi input; vj input
function [out_i, E_cable, out_j]= cable(k_cable,l_cable,xi,xj,c,vi,vj)
% damp and D are initialized as zero
damp = 0;
D = 0;

% Node distance
x = xj-xi;
dist = norm(x);

% Only when the cable is in tension there is non-zero force and damping
if  dist-l_cable > 0
    D = dist-l_cable;
    v = vj - vi;
    damp = -c*dot(v,x)/dist^2;
end

% Forces on the end nodes
out_i = k_cable*D*(x)/dist - damp*(x);
out_j = -k_cable*D*(x)/dist + damp*(x);

% Energy stored in the cable
E_cable = 0.5*k_cable*D^2;
end

== matlab function Kinematic_Model_Simulink/24 cables/cable 10--11 ==
  data: out_i output; E_cable output; out_j output; k_cable input; l_cable input; xi input; xj input; c input; vi input; vj input
function [out_i, E_cable, out_j]= cable(k_cable,l_cable,xi,xj,c,vi,vj)
% damp and D are initialized as zero
damp = 0;
D = 0;

% Node distance
x = xj-xi;
dist = norm(x);

% Only when the cable is in tension there is non-zero force and damping
if  dist-l_cable > 0
    D = dist-l_cable;
    v = vj - vi;
    damp = -c*dot(v,x)/dist^2;
end

% Forces on the end nodes
out_i = k_cable*D*(x)/dist - damp*(x);
out_j = -k_cable*D*(x)/dist + damp*(x);

% Energy stored in the cable
E_cable = 0.5*k_cable*D^2;
end

== matlab function Kinematic_Model_Simulink/24 cables/cable 11--12 ==
  data: out_i output; E_cable output; out_j output; k_cable input; l_cable input; xi input; xj input; c input; vi input; vj input
function [out_i, E_cable, out_j]= cable(k_cable,l_cable,xi,xj,c,vi,vj)
% damp and D are initialized as zero
damp = 0;
D = 0;

% Node distance
x = xj-xi;
dist = norm(x);

% Only when the cable is in tension there is non-zero force and damping
if  dist-l_cable > 0
    D = dist-l_cable;
    v = vj - vi;
    damp = -c*dot(v,x)/dist^2;
end

% Forces on the end nodes
out_i = k_cable*D*(x)/dist - damp*(x);
out_j = -k_cable*D*(x)/dist + damp*(x);

% Energy stored in the cable
E_cable = 0.5*k_cable*D^2;
end

== matlab function Kinematic_Model_Simulink/24 cables/cable 5--8 ==
  data: out_i output; E_cable output; out_j output; k_cable input; l_cable input; xi input; xj input; c input; vi input; vj input
function [out_i, E_cable, out_j]= cable(k_cable,l_cable,xi,xj,c,vi,vj)
% damp and D are initialized as zero
damp = 0;
D = 0;

% Node distance
x = xj-xi;
dist = norm(x);

% Only when the cable is in tension there is non-zero force and damping
if  dist-l_cable > 0
    D = dist-l_cable;
    v = vj - vi;
    damp = -c*dot(v,x)/dist^2;
end

% Forces on the end nodes
out_i = k_cable*D*(x)/dist - damp*(x);
out_j = -k_cable*D*(x)/dist + damp*(x);

% Energy stored in the cable
E_cable = 0.5*k_cable*D^2;
end

== matlab function Kinematic_Model_Simulink/24 cables/cable 5--7 ==
  data: out_i output; E_cable output; out_j output; k_cable input; l_cable input; xi input; xj input; c input; vi input; vj input
function [out_i, E_cable, out_j]= cable(k_cable,l_cable,xi,xj,c,vi,vj)
% damp and D are initialized as zero
damp = 0;
D = 0;

% Node distance
x = xj-xi;
dist = norm(x);

% Only when the cable is in tension there is non-zero force and damping
if  dist-l_cable > 0
    D = dist-l_cable;
    v = vj - vi;
    damp = -c*dot(v,x)/dist^2;
end

% Forces on the end nodes
out_i = k_cable*D*(x)/dist - damp*(x);
out_j = -k_cable*D*(x)/dist + damp*(x);

% Energy stored in the cable
E_cable = 0.5*k_cable*D^2;
end

== matlab function Kinematic_Model_Simulink/24 cables/cable 5--12 ==
  data: out_i output; E_cable output; out_j output; k_cable input; l_cable input; xi input; xj input; c input; vi input; vj input
function [out_i, E_cable, out_j]= cable(k_cable,l_cable,xi,xj,c,vi,vj)
% damp and D are initialized as zero
damp = 0;
D = 0;

% Node distance
x = xj-xi;
dist = norm(x);

% Only when the cable is in tension there is non-zero force and damping
if  dist-l_cable > 0
    D = dist-l_cable;
    v = vj - vi;
    damp = -c*dot(v,x)/dist^2;
end

% Forces on the end nodes
out_i = k_cable*D*(x)/dist - damp*(x);
out_j = -k_cable*D*(x)/dist + damp*(x);

% Energy stored in the cable
E_cable = 0.5*k_cable*D^2;
end
